simulink library "Steer_Ackermann"  (R2025b)
settings: Solver=VariableStepAuto  StartTime=0.0  StopTime=10.0  RelTol=1e-3
undefined symbols (not defined in the file): Susp
libraries: Steer_Ackermann_Driver x1, Steer_Ackermann_WheelsOnly x1, Steer_DriverWheel x1, Steer_LUT_Driver x1, Steer_Ackermann_None x1, Steer_Control_Axle2 x1
Description:
  | Component of Simscape Vehicle Templates Library
  | 
  | Copyright 2018-2024 The MathWorks, Inc.
settings Model: Creator=smiller  LastModifiedBy=smiller
settings SolverCC: AlgebraicLoopSolver=TrustRegion
settings DataIOCC: ReturnWorkspaceOutputs=off
settings DebuggingCC: UnconnectedInputMsg=warning  UnconnectedOutputMsg=warning  UnconnectedLineMsg=warning  ArithmeticOperatorsInVariantConditions=warning
settings ModelReferenceCC: EnableRefExpFcnMdlSchedulingChecks=on
settings SFSimCC: CustomCodeUndefinedFunction=UseInterfaceOnly
settings RTWCC: GPUComputeCapability=3.5  DLArmComputeVersion=19.05

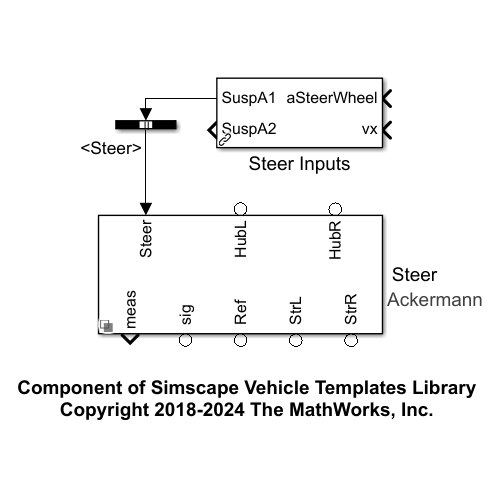
[thumbnail: Simulink's stored preview of the top-level diagram]
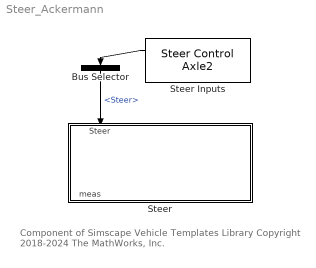
== system Steer_Ackermann ==
  note: Component of Simscape Vehicle Templates Library
      | Copyright 2018-2024 The MathWorks, Inc.
  Bus Selector : BusSelector  OutputSignals=Steer
  Steer : Subsystem  Variant=on  VariantControlMode=label  VariantControl=Variant1  LabelModeActiveChoice=Ackermann  mask{Steer=Susp.Steer, VariantLabel=Susp.Steer.class.Value}
      mask prompts: Steer "Steer Parameters"; VariantLabel "Variant Label"
      mask init:
      | curblk = gcb;
      | 
      | % Set variant for this subsystem
      | set_param(curblk,'LabelModeActiveChoice',VariantLabel);
      settings: AttributesFormatString=%<ActiveVariant>
      mask Display: disp(' ')
  Steer Inputs : Steer_Control_Axle2/Steer Control Axle2  Steer=Control.Default.Steer
  wires:
  Steer Inputs/1 -> Bus Selector/1
  Bus Selector/1 -> Steer/1(Steer)  "<Steer>"

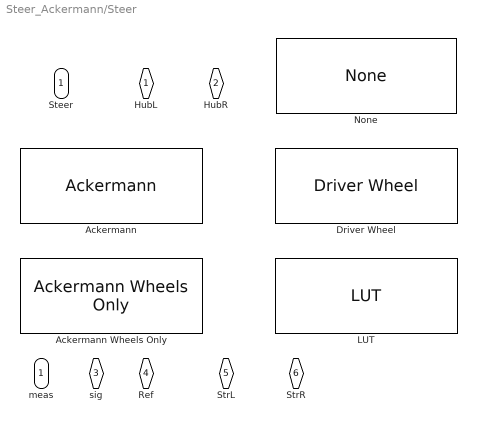
== system Steer_Ackermann/Steer ==
  Steer : Inport
  Ackermann : Steer_Ackermann_Driver/Ackermann  VariantControl=Ackermann  hp_wheel=Steer.Wheel.sMount.Value  wheel_axis_incl=Steer.Wheel.aAxis.Value  Wheel=Steer.Wheel  whl2rack_filter=1/Steer.Rack.fActuatorCutoff.Value  yTrack=Steer.xTrack.Value  xwheelbase=Steer.xWheelbase.Value  steer_ratio=Susp.Steer.rSteer.Value  aCaster=Steer.aCaster.Value  aKPI=Steer.aKPI.Value  clr_wheel=Visual.SteeringWheel.clr  opc_wheel=Visual.part.opc  DriverHuman=Steer.DriverHuman
  Ackermann Wheels Only : Steer_Ackermann_WheelsOnly/Ackermann Wheels Only  VariantControl=AckermannWheelsOnly  whl2rack_filter=1/Steer.Rack.fActuatorCutoff.Value  yTrack=Steer.xTrack.Value  xwheelbase=Steer.xWheelbase.Value  steer_ratio=Susp.Steer.rSteer.Value  aCaster=Steer.aCaster.Value  aKPI=Steer.aKPI.Value
  Driver Wheel : Steer_DriverWheel/Driver Wheel  VariantControl=DriverWheel  hp_wheel=Steer.Wheel.sMount.Value  wheel_axis_incl=Steer.Wheel.aAxis.Value  Wheel=Steer.Wheel  whl2rack_filter=1/Steer.Rack.fActuatorCutoff.Value  clr_wheel=Visual.SteeringWheel.clr  opc_wheel=Visual.part.opc  DriverHuman=Steer.DriverHuman
  LUT : Steer_LUT_Driver/LUT  VariantControl=LUT  aStrWhl=Steer.Ratio.aWhl.Value  aToeL=Steer.Ratio.aToeL.Value  aToeR=Steer.Ratio.aToeR.Value  hp_wheel=Steer.Wheel.sMount.Value  wheel_axis_incl=Steer.Wheel.aAxis.Value  Wheel=Steer.Wheel  whl2rack_filter=1/Steer.Rack.fActuatorCutoff.Value  aCaster=Steer.aCaster.Value  aKPI=Steer.aKPI.Value  clr_wheel=Visual.SteeringWheel.clr  opc_wheel=Visual.part.opc  DriverHuman=Steer.DriverHuman
  None : Steer_Ackermann_None/None  SystemSampleTime=-1  VariantControl=None  VariantActivationTime=update diagram  Latency=0  AutoFrameSizeCalculation=off
  " HubL" : PMIOPort  Side=Left
  " HubR" : PMIOPort  Port=2  Side=Left
  " sig" : PMIOPort  Port=3  Side=Right
  " Ref" : PMIOPort  Port=4  Side=Right
  " StrL" : PMIOPort  Port=5  Side=Right
  " StrR" : PMIOPort  Port=6  Side=Right
  meas : Outport  VectorParamsAs1DForOutWhenUnconnected=off
